simulink model "Sim_Model_2ndODE_ex1"  (Simulink 8.0)
settings: Solver=ode45  StartTime=0.0  StopTime=10.0  RelTol=1e-3
settings Model: Creator=David  LastModifiedBy=David
settings DataIOCC: SignalLoggingSaveFormat=ModelDataLogs
settings DebuggingCC: FcnCallInpInsideContextMsg=UseLocalSettings
settings GRTTargetCC: CombineOutputUpdateFcns=off  GRTInterface=on

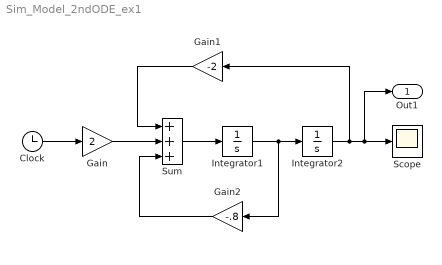
== system Sim_Model_2ndODE_ex1 ==
  Clock : Clock
  Gain : Gain  Gain=2
  Gain1 : Gain  Gain=-2
  Gain2 : Gain  Gain=-.8
  Integrator1 : Integrator  InitialCondition=2
  Integrator2 : Integrator  InitialCondition=1
  Scope : Scope
  Sum : Sum  Inputs=+++
  Out1 : Outport
  wires:
  Clock/1 -> Gain/1
  Sum/1 -> Integrator1/1
  Gain1/1 -> Sum/1
  Gain/1 -> Sum/2
  Integrator1/1 -> Gain2/1, Integrator2/1
  Integrator2/1 -> Gain1/1, Out1/1, Scope/1
  Gain2/1 -> Sum/3
